simulink model "ascensore_modello_simulink"  (R2014b)
settings: Solver=ode45  StartTime=0.0  StopTime=10.0  RelTol=1e-3
values from neighbouring files (symbols this model uses):
  C = 100    [ascensore_workspace_matlab.mat]    (also in parametri_modello_ascensore.m)
  g = 9.81    [ascensore_workspace_matlab.mat]    (also in parametri_modello_ascensore.m)
  J = 10    [ascensore_workspace_matlab.mat]    (also in parametri_modello_ascensore.m)
  K = 500    [ascensore_workspace_matlab.mat]    (also in parametri_modello_ascensore.m)
  m = 500    [ascensore_workspace_matlab.mat]    (also in parametri_modello_ascensore.m)
  M = 1000    [ascensore_workspace_matlab.mat]    (also in parametri_modello_ascensore.m)
  R = 0.25    [ascensore_workspace_matlab.mat]    (also in parametri_modello_ascensore.m)
settings Model: Creator=ivo-chan  LastModifiedBy=ivo-chan

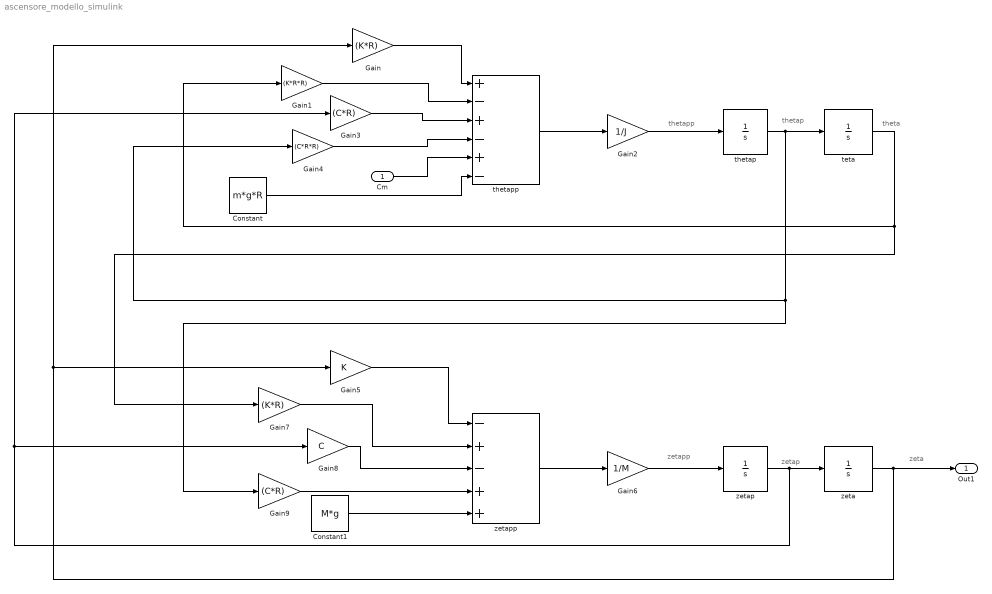
== system ascensore_modello_simulink ==
  note: zeta
  note: zetap
  note: zetapp
  note: theta
  note: thetap
  note: thetapp
  Cm : Inport
  Constant : Constant  Value=m*g*R
  Constant1 : Constant  Value=M*g
  Gain : Gain  Gain=(K*R)
  Gain1 : Gain  Gain=(K*R*R)
  Gain2 : Gain  Gain=1/J
  Gain3 : Gain  Gain=(C*R)
  Gain4 : Gain  Gain=(C*R*R)
  Gain5 : Gain  Gain=K
  Gain6 : Gain  Gain=1/M
  Gain7 : Gain  Gain=(K*R)
  Gain8 : Gain  Gain=C
  Gain9 : Gain  Gain=(C*R)
  teta : Integrator
  thetap : Integrator
  thetapp : Sum  Inputs=+-+-+-
  zeta : Integrator
  zetap : Integrator
  zetapp : Sum  Inputs=-+-++
  Out1 : Outport
  wires:
  Gain/1 -> thetapp/1
  thetapp/1 -> Gain2/1
  Gain1/1 -> thetapp/2
  Gain3/1 -> thetapp/3
  Gain4/1 -> thetapp/4
  Cm/1 -> thetapp/5
  Constant/1 -> thetapp/6
  Gain2/1 -> thetap/1
  thetap/1 -> Gain9/1, Gain4/1, teta/1
  teta/1 -> Gain1/1, Gain7/1
  Gain5/1 -> zetapp/1
  zetapp/1 -> Gain6/1
  Gain7/1 -> zetapp/2
  Gain8/1 -> zetapp/3
  Gain9/1 -> zetapp/4
  Constant1/1 -> zetapp/5
  Gain6/1 -> zetap/1
  zetap/1 -> Gain3/1, Gain8/1, zeta/1
  zeta/1 -> Gain/1, Gain5/1, Out1/1
